simulink model "Lightning_McSeas_VCU"  (R2021b)
settings: Solver=FixedStepDiscrete  StartTime=0.0  StopTime=10.0  FixedStep=0.01  RelTol=1e-3  EnableMultiTasking=on
PreLoadFcn:
  | try, model_open; catch, disp('Error occurred while executing model pre-load callback: model_open.m'); disp('Please assure that the MATLAB working directory is set to the model directory before opening.'); end
InitFcn:
  | try, model_open; catch, end
undefined symbols (not defined in the file): dataName, enumName, enumValue, GCM, raptor_get_safe_string
libraries: Raptor_lib x67, simulink x8
(part 3 of 3)

== system Lightning_McSeas_VCU/Foreground/CAN/RC Rx/MCU/If statement for on off switch4 ==
  value in : Inport
  Constant2 : Constant
  Constant3 : Constant  Value=0
  If : If  IfExpression=u1 >250
  If Action Subsystem : Subsystem  TreatAsAtomicUnit=on
  If Action Subsystem1 : Subsystem  TreatAsAtomicUnit=on
  Merge : Merge
  Value out : Outport
  wires:
  value in/1 -> If/1
  Constant2/1 -> If Action Subsystem/1(Xa)
  If Action Subsystem1/1(Out1) -> Merge/2
  Merge/1 -> Value out/1
  If/1 -> If Action Subsystem/Action
  Constant3/1 -> If Action Subsystem1/1(Xb)
  If Action Subsystem/1(Out1) -> Merge/1
  If/2 -> If Action Subsystem1/Action

== system Lightning_McSeas_VCU/Foreground/CAN/RC Rx/MCU/If statement for on off switch5 ==
  Contact value : Inport
  Add : Sum
  If : If  IfExpression=u1 < 1
  If Action Subsystem1 : Subsystem  TreatAsAtomicUnit=on
  If Action Subsystem3 : Subsystem  TreatAsAtomicUnit=on
  Value out : Outport
  wires:
  If/2 -> If Action Subsystem1/Action
  Contact value/1 -> If Action Subsystem1/1(Xb1), If Action Subsystem3/1(Xb1), If/1
  If Action Subsystem1/1(Out1) -> Add/2
  Add/1 -> Value out/1
  If/1 -> If Action Subsystem3/Action
  If Action Subsystem3/1(Out1) -> Add/1

== system Lightning_McSeas_VCU/Foreground/CAN/RC Rx/MCU/Left Motor ==
  Throttle : Inport
  Rudder : Inport  Port=2
  Drive Mode : Inport  Port=3
  If statement for on off switch1 : Subsystem
  Sum : Sum  Inputs=|+-
  Value out : Outport
  wires:
  Throttle/1 -> Sum/1
  Sum/1 -> If statement for on off switch1/2(Throttle)
  Rudder/1 -> Sum/2
  Drive Mode/1 -> If statement for on off switch1/1(Drive Mode swtich)
  If statement for on off switch1/1(Value out) -> Value out/1

== system Lightning_McSeas_VCU/Foreground/CAN/RC Rx/MCU/Right Motor ==
  Throttle : Inport
  Rudder : Inport  Port=2
  Drive Mode : Inport  Port=3
  Constant : Constant  Value=-1
  If statement for on off switch1 : Subsystem
  Product : Product
  Sum : Sum  Inputs=|+-
  Value out : Outport
  wires:
  Throttle/1 -> Sum/1
  Sum/1 -> If statement for on off switch1/2(Throttle)
  Rudder/1 -> Sum/2
  Drive Mode/1 -> If statement for on off switch1/1(Drive Mode swtich)
  If statement for on off switch1/1(Value out) -> Product/1
  Product/1 -> Value out/1
  Constant/1 -> Product/2

== system Lightning_McSeas_VCU/GCM48 Power Up_Down/Background/Wake sources/Debounce2/SetRst Init = 0 ==
  Set : Inport
  Rst : Inport  Port=2
  Constant : Constant  Value=boolean(0)
  Constant1 : Constant  Value=boolean(1)
  Multiport Switch : MultiPortSwitch  DataPortOrder=Zero-based contiguous  Inputs=2  zeroidx=on
  Multiport Switch1 : MultiPortSwitch  DataPortOrder=Zero-based contiguous  Inputs=2  zeroidx=on
  Unit Delay : UnitDelay  InitialCondition=init  SampleTime=-1  HasFrameUpgradeWarning=on
  Bool : Outport  VectorParamsAs1DForOutWhenUnconnected=off
  wires:
  Multiport Switch1/1 -> Multiport Switch/2
  Constant1/1 -> Multiport Switch1/3
  Constant/1 -> Multiport Switch/3
  Rst/1 -> Multiport Switch/1
  Set/1 -> Multiport Switch1/1
  Multiport Switch/1 -> Bool/1, Unit Delay/1
  Unit Delay/1 -> Multiport Switch1/2

== system Lightning_McSeas_VCU/GCM48 Power Up_Down/Background/Wake sources/Decode amd Ignore Some Wake Sources/Startup Wake Source ==
  Wake_SourceBitAndWakeConfigRegister : Inport
  Enable : EnablePort
  raptor_measurement : Raptor_lib/Data Storage/raptor_measurement  paramName='WakeSource_Startup'  nameSource=Parameter  calDispType=Number  calEnum={'False', 'True'}  calGain=1.0  calOffset=0.0  calMax=inf  calMin=-inf  calFormat='-1'  calUnit=''  calHelp=''  calAccess=4  calFunction=group  calVisible=on
      settings: SourceProductName=Raptor
  wires:
  Wake_SourceBitAndWakeConfigRegister/1 -> raptor_measurement/1

== system Lightning_McSeas_VCU/Foreground/CAN/RC Rx/Actuators/If statement for on off switch1/If Action Subsystem ==
  Xa : Inport
  Action Port : ActionPort
  Out1 : Outport
  wires:
  Xa/1 -> Out1/1

== system Lightning_McSeas_VCU/Foreground/CAN/RC Rx/Actuators/If statement for on off switch1/If Action Subsystem1 ==
  Xb : Inport
  Action Port : ActionPort
  Out1 : Outport
  wires:
  Xb/1 -> Out1/1

== system Lightning_McSeas_VCU/Foreground/CAN/RC Rx/Actuators/If statement for on off switch1/If Action Subsystem2 ==
  Xb : Inport
  Action Port : ActionPort
  Out1 : Outport
  wires:
  Xb/1 -> Out1/1

== system Lightning_McSeas_VCU/Foreground/CAN/RC Rx/Battery Switch/If statement for on off switch/If Action Subsystem ==
  Xa : Inport
  Action Port : ActionPort  ActionPortLabel=if(u1 > 1200)
  Out1 : Outport
  wires:
  Xa/1 -> Out1/1

== system Lightning_McSeas_VCU/Foreground/CAN/RC Rx/Battery Switch/If statement for on off switch/If Action Subsystem1 ==
  Xb : Inport
  Action Port : ActionPort  ActionPortLabel=else
  Out1 : Outport
  wires:
  Xb/1 -> Out1/1

== system Lightning_McSeas_VCU/Foreground/CAN/RC Rx/Battery Switch/If statement for on off switch1/If Action Subsystem ==
  Xa : Inport
  Action Port : ActionPort  ActionPortLabel=if(u1 > 1200)
  Out1 : Outport
  wires:
  Xa/1 -> Out1/1

== system Lightning_McSeas_VCU/Foreground/CAN/RC Rx/Battery Switch/If statement for on off switch1/If Action Subsystem1 ==
  Xb : Inport
  Action Port : ActionPort  ActionPortLabel=else
  Out1 : Outport
  wires:
  Xb/1 -> Out1/1

== system Lightning_McSeas_VCU/Foreground/CAN/RC Rx/Battery Switch/If statement for on off switch2/If Action Subsystem ==
  Xa : Inport
  Action Port : ActionPort  ActionPortLabel=if(u1 > 250)
  Out1 : Outport
  wires:
  Xa/1 -> Out1/1

== system Lightning_McSeas_VCU/Foreground/CAN/RC Rx/Battery Switch/If statement for on off switch2/If Action Subsystem1 ==
  Xb : Inport
  Action Port : ActionPort  ActionPortLabel=else
  Out1 : Outport
  wires:
  Xb/1 -> Out1/1

== system Lightning_McSeas_VCU/Foreground/CAN/RC Rx/MCU/If statement for on off switch1/If Action Subsystem ==
  Xa : Inport
  Action Port : ActionPort  ActionPortLabel=if(u1 > 1200)
  Out1 : Outport
  wires:
  Xa/1 -> Out1/1

== system Lightning_McSeas_VCU/Foreground/CAN/RC Rx/MCU/If statement for on off switch1/If Action Subsystem1 ==
  Xb : Inport
  Action Port : ActionPort  ActionPortLabel=else
  Out1 : Outport
  wires:
  Xb/1 -> Out1/1

== system Lightning_McSeas_VCU/Foreground/CAN/RC Rx/MCU/If statement for on off switch2/If Action Subsystem1 ==
  Xb : Inport
  Xb1 : Inport  Port=2
  Action Port : ActionPort
  Product : Product
  Out1 : Outport
  wires:
  Xb/1 -> Product/2
  Xb1/1 -> Product/1
  Product/1 -> Out1/1

== system Lightning_McSeas_VCU/Foreground/CAN/RC Rx/MCU/If statement for on off switch2/If Action Subsystem2 ==
  Xb : Inport
  Action Port : ActionPort  ActionPortLabel=elseif(u1>250)
  Out1 : Outport
  wires:
  Xb/1 -> Out1/1

== system Lightning_McSeas_VCU/Foreground/CAN/RC Rx/MCU/If statement for on off switch2/If Action Subsystem3 ==
  Xb : Inport
  Action Port : ActionPort  ActionPortLabel=if(u1 > 1200)
  Out1 : Outport
  wires:
  Xb/1 -> Out1/1

== system Lightning_McSeas_VCU/Foreground/CAN/RC Rx/MCU/If statement for on off switch2/If Action Subsystem4 ==
  Xb : Inport
  Action Port : ActionPort  ActionPortLabel=else
  Out1 : Outport
  wires:
  Xb/1 -> Out1/1

== system Lightning_McSeas_VCU/Foreground/CAN/RC Rx/MCU/If statement for on off switch3/If Action Subsystem1 ==
  Xb : Inport
  Xb1 : Inport  Port=2
  Action Port : ActionPort
  Product : Product
  Out1 : Outport
  wires:
  Xb/1 -> Product/2
  Xb1/1 -> Product/1
  Product/1 -> Out1/1

== system Lightning_McSeas_VCU/Foreground/CAN/RC Rx/MCU/If statement for on off switch3/If Action Subsystem2 ==
  Xb : Inport
  Action Port : ActionPort
  Out1 : Outport
  wires:
  Xb/1 -> Out1/1

== system Lightning_McSeas_VCU/Foreground/CAN/RC Rx/MCU/If statement for on off switch3/If Action Subsystem3 ==
  Xb : Inport
  Xb1 : Inport  Port=2
  Action Port : ActionPort
  Product : Product
  Out1 : Outport
  wires:
  Xb/1 -> Product/2
  Xb1/1 -> Product/1
  Product/1 -> Out1/1

== system Lightning_McSeas_VCU/Foreground/CAN/RC Rx/MCU/If statement for on off switch4/If Action Subsystem ==
  Xa : Inport
  Action Port : ActionPort  ActionPortLabel=if(u1 >250)
  Out1 : Outport
  wires:
  Xa/1 -> Out1/1

== system Lightning_McSeas_VCU/Foreground/CAN/RC Rx/MCU/If statement for on off switch4/If Action Subsystem1 ==
  Xb : Inport
  Action Port : ActionPort  ActionPortLabel=else
  Out1 : Outport
  wires:
  Xb/1 -> Out1/1

== system Lightning_McSeas_VCU/Foreground/CAN/RC Rx/MCU/If statement for on off switch5/If Action Subsystem1 ==
  Xb1 : Inport
  Action Port : ActionPort
  Out1 : Outport
  wires:
  Xb1/1 -> Out1/1

== system Lightning_McSeas_VCU/Foreground/CAN/RC Rx/MCU/If statement for on off switch5/If Action Subsystem3 ==
  Xb1 : Inport
  Action Port : ActionPort
  Transport Delay : TransportDelay  DelayTime=0.5
  Out1 : Outport
  wires:
  Xb1/1 -> Transport Delay/1
  Transport Delay/1 -> Out1/1

== system Lightning_McSeas_VCU/Foreground/CAN/RC Rx/MCU/Left Motor/If statement for on off switch1 ==
  Drive Mode swtich : Inport
  Throttle : Inport  Port=2
  Add : Sum  Inputs=+++
  Constant3 : Constant  Value=0
  If : If  IfExpression=u1 > 1400  ElseIfExpressions=u1<250
  If Action Subsystem : Subsystem  TreatAsAtomicUnit=on
  If Action Subsystem1 : Subsystem  TreatAsAtomicUnit=on
  If Action Subsystem2 : Subsystem  TreatAsAtomicUnit=on
  Value out : Outport
  wires:
  If Action Subsystem1/1(Out1) -> Add/2
  Add/1 -> Value out/1
  If/1 -> If Action Subsystem/Action
  Constant3/1 -> If Action Subsystem1/1(Xb)
  If Action Subsystem/1(Out1) -> Add/1
  If/3 -> If Action Subsystem1/Action
  Drive Mode swtich/1 -> If/1
  If/2 -> If Action Subsystem2/Action
  If Action Subsystem2/1(Out1) -> Add/3
  Throttle/1 -> If Action Subsystem2/1(Xa), If Action Subsystem/1(Xa)

== system Lightning_McSeas_VCU/Foreground/CAN/RC Rx/MCU/Right Motor/If statement for on off switch1 ==
  Drive Mode swtich : Inport
  Throttle : Inport  Port=2
  Add : Sum  Inputs=+++
  Constant3 : Constant  Value=0
  If : If  IfExpression=u1 > 1400  ElseIfExpressions=u1<250
  If Action Subsystem : Subsystem  TreatAsAtomicUnit=on
  If Action Subsystem1 : Subsystem  TreatAsAtomicUnit=on
  If Action Subsystem2 : Subsystem  TreatAsAtomicUnit=on
  Value out : Outport
  wires:
  If Action Subsystem1/1(Out1) -> Add/2
  Add/1 -> Value out/1
  If/1 -> If Action Subsystem/Action
  Constant3/1 -> If Action Subsystem1/1(Xb)
  If Action Subsystem/1(Out1) -> Add/1
  If/3 -> If Action Subsystem1/Action
  Drive Mode swtich/1 -> If/1
  If/2 -> If Action Subsystem2/Action
  If Action Subsystem2/1(Out1) -> Add/3
  Throttle/1 -> If Action Subsystem2/1(Xa), If Action Subsystem/1(Xa)

== system Lightning_McSeas_VCU/Foreground/CAN/RC Rx/MCU/Left Motor/If statement for on off switch1/If Action Subsystem ==
  Xa : Inport
  Action Port : ActionPort  ActionPortLabel=if(u1 > 1400)
  Out1 : Outport
  wires:
  Xa/1 -> Out1/1

== system Lightning_McSeas_VCU/Foreground/CAN/RC Rx/MCU/Left Motor/If statement for on off switch1/If Action Subsystem1 ==
  Xb : Inport
  Action Port : ActionPort  ActionPortLabel=else
  Out1 : Outport
  wires:
  Xb/1 -> Out1/1

== system Lightning_McSeas_VCU/Foreground/CAN/RC Rx/MCU/Left Motor/If statement for on off switch1/If Action Subsystem2 ==
  Xa : Inport
  Action Port : ActionPort  ActionPortLabel=elseif(u1<250)
  Constant : Constant  Value=-1
  Product : Product
  Out1 : Outport
  wires:
  Xa/1 -> Product/1
  Product/1 -> Out1/1
  Constant/1 -> Product/2

== system Lightning_McSeas_VCU/Foreground/CAN/RC Rx/MCU/Right Motor/If statement for on off switch1/If Action Subsystem ==
  Xa : Inport
  Action Port : ActionPort  ActionPortLabel=if(u1 > 1400)
  Out1 : Outport
  wires:
  Xa/1 -> Out1/1

== system Lightning_McSeas_VCU/Foreground/CAN/RC Rx/MCU/Right Motor/If statement for on off switch1/If Action Subsystem1 ==
  Xb : Inport
  Action Port : ActionPort  ActionPortLabel=else
  Out1 : Outport
  wires:
  Xb/1 -> Out1/1

== system Lightning_McSeas_VCU/Foreground/CAN/RC Rx/MCU/Right Motor/If statement for on off switch1/If Action Subsystem2 ==
  Xa : Inport
  Action Port : ActionPort  ActionPortLabel=elseif(u1<250)
  Constant : Constant  Value=-1
  Product : Product
  Out1 : Outport
  wires:
  Xa/1 -> Product/1
  Product/1 -> Out1/1
  Constant/1 -> Product/2
